simulink model "rti1401_program_controls_2018"  (R2017b)
settings: Solver=ode1  StartTime=0.0  StopTime=Inf  FixedStep=0.001  RelTol=1e-3  EnableMultiTasking=on
PreLoadFcn:
  | dataCar
  | load_vars
  | structAero
  | structEstimPar
  | structSensors
  | structSettings
PostLoadFcn:
  | , if any(exist('dsrtsu_mdlpostloadfcn', 'file') == [2, 3, 6]), try dsrtsu_mdlpostloadfcn('Execute', bdroot); catch fprintf('Error in PostLoadFcn (dsrtsu_mdlpostloadfcn) for model "%s":\n %s\n', bdroot, lasterr); end, end,
InitFcn:
  | dataCar
  | load_vars
  | structAero
  | structEstimPar
  | structSensors
  | structSettings
StartFcn:
  | dataCar
  | load_vars
  | structAero
  | structEstimPar
  | structSensors
  | structSettings
values from neighbouring files (symbols this model uses):
  Throttle_limits = [0.15, 0.90, 0.16, 0.92]    [load_vars.m]
undefined symbols (not defined in the file or in its folder): car, sensors, tau
libraries: rtican x44, hdlsllib x32, simulink x8, rti1401lib_II_base x1
(part 5 of 11)

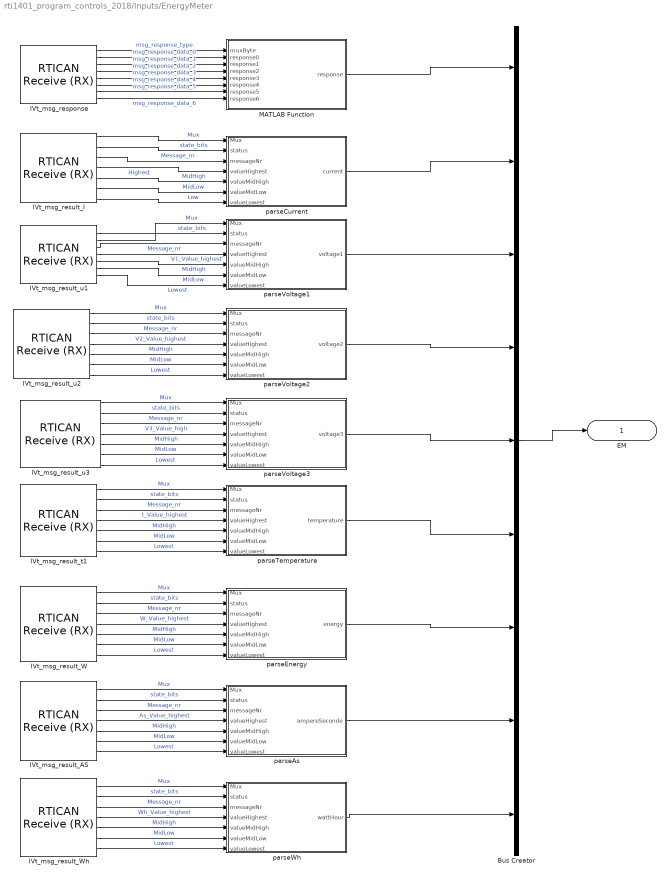
== system rti1401_program_controls_2018/Inputs/EnergyMeter ==
  Bus Creator : BusCreator  Inputs=9
  IVt_msg_response : rtican/RTICAN Receive (RX)   Reserved1=[]  Reserved2=[]  Reserved3=[]  Reserved4=[]  SfcnMessage=[]  Msg_Struct=[]  BoardTypeNo=[]  BoardNo=[]  ChannelNo=[]  Parameters=[]  DialogFcn=[]  UnitName=[]  Revision=[]  UnitValues=[]  DSProperties=struct('RTI',struct('Version',uint32(5),'BlockType',struct('isSLSource',uint8(1),'isSLSink',uint8(1),'isHWSource',uint8(0),'isHWSink',uint8(0),'isSetup',uint8(0),'isInline',uint8(1),'isNonInline',uint8(0),'isInterrupt',uint8(0),'isChannelwise',uint8(0)),'IOBoardType','RTICAN','UnitType','MESSAGE','Identifier','RX','DialogType','MSVC','BlockSet','RTICAN','SlaveProcessor','CAN'))  RTIBlockInterface=struct('OutputPortsWidth',int32([1 1 1 1 1 1 1 1]),'OutputPortsActive',[1 1 1 1 1 1 1 1],'OutputPortsName',{{'msg_response_type','msg_response_data_0','msg_response_data_1','msg_response_data_2','msg_response_data_3','msg_response_data_4','msg_response_data_5','msg_response_data_6'}},'OutputPortsDataType',{{'SS_UINT8','SS_UINT8','SS_UINT8','SS_UINT8','SS_UINT8','SS_UINT8','SS_UINT8','SS_UINT8'}},'OutputPortsLabel',{{'msg_response_type','msg_response_data_0','msg_response_data_1','msg_response_data_2','msg_response_data_3','msg_response_data_4','msg_response_data_5','msg_response_data_6'}},'OutputPortsLabelMode','ON','InputPortsWidth',int32(0),'InputPortsActive',0,'DialogFcn','rtican_message_interface_gui','BlockDisplay',{{'','center'}},'IconTransparency','on','ParameterTunableNames',{{}},'InitLevel',3,'BlockName',struct('Token',{{'IVt_msg_response'}}),'SampleTime',{{-1}},'TriggerPort',{{'none'}},'EnablePort',{{'none'}})  RTIBlockParameters=struct('BoardTypeNo',{{1,'OFF',[]}},'BoardNo',{{2,'ON',[1 16]}},'ChannelNo',{{2,'ON',[1 2]}},'Parameters',{{struct('DataFileSupport',struct('DataFileSelectedMaster',0,'DataFileSelectedLocal',0,'DataFileName',['<no datafile support>|'],'DataFileDate','','SelectedFile',['<no file selected>']),'Options',struct('StatusSelected',0,'TimeSelected',0,'DeltaTimeSelected',0,'BytePortSelected',0,'MessageLengthSelected',0,'TriggerPort',struct('Selected',0,'TriggerType',0),'UserCoding',struct('Selected',0,'InterfaceFile','UserDecodingFile','FcnName','UserDecodeFcn','InportSelected',0,'InportWidth',1,'OutportSelected',0,'OutportWidth',1),'EnablePortSelected',0,'SignalOnPortnameSelected',1,'UseRXService',0),'Message',struct('MsgOnBlocknameSelected',1,'MsgName','IVt_msg_response','MsgIdFormat',0,'MsgId',1297,'MsgLength',8,'NumSignals',8,'SampleTime',-1,'Signal',struct('SgnName',{'msg_response_type','msg_response_data_0','msg_response_data_1','msg_response_data_2','msg_response_data_3','msg_response_data_4','msg_response_data_5','msg_response_data_6'},'SgnStartBit',{0,8,16,24,32,40,48,56},'SgnLength',{8,8,8,8,8,8,8,8},'SgnType',{0,0,0,0,0,0,0,0},'ModeValue',{-1,-1,-1,-1,-1,-1,-1,-1},'DataType',{0,0,0,0,0,0,0,0},'ByteLayout',{1,1,1,1,1,1,1,1},'Factor',{1,1,1,1,1,1,1,1},'Offset',{0,0,0,0,0,0,0,0},'SgnComment',{{''},{''},{''},{''},{''},{''},{''},{''}},'SgnUnit',{'','','','','','','',''},'Min',{0,0,0,0,0,0,0,0},'Max',{255,255,255,255,255,255,255,255},'SLDataType',{'SS_UINT8','SS_UINT8','SS_UINT8','SS_UINT8','SS_UINT8','SS_UINT8','SS_UINT8','SS_UINT8'}),'MsgIdNumFormat',1,'MsgComment',{{''}}),'Version',1.2,'general',struct('isFromLib',0)),'OFF',[]}},'GroupId',{{struct('Group',{{'RTICAN'}},'No',4,'Behavior',{{'NAMECHANGE'}},'BlockType',{{'SINK'}},'NameChangeFlag',0),'OFF',[]}},'SFcnRTICANMessage',{{struct('MsgType','RX','SFcnPortType','Scalar','MsgName','IVt_msg_response','MsgIdFormat','STD','MsgId',1297,'MsgLength',8,'NumSignals',8,'SampleTime',-1,'Signal',struct('SgnName',{'msg_response_type','msg_response_data_0','msg_response_data_1','msg_response_data_2','msg_response_data_3','msg_response_data_4','msg_response_data_5','msg_response_data_6'},'SgnStartBit',{0,8,16,24,32,40,48,56},'SgnLength',{8,8,8,8,8,8,8,8},'SgnType',{'standard','standard','standard','standard','standard','standard','standard','standard'},'ModeValue',{-1,-1,-1,-1,-1,-1,-1,-1},'DataType',{['unsigned int'],['unsigned int'],['unsigned int'],['unsigned int'],['unsigned int'],['unsigned int'],['unsigned int'],['unsigned int']},'ByteLayout',{['big endian'],['big endian'],['big endian'],['big endian'],['big endian'],['big endian'],['big endian'],['big endian']},'Factor',{1,1,1,1,1,1,1,1},'Offset',{0,0,0,0,0,0,0,0},'SLDataType',{'SS_UINT8','SS_UINT8','SS_UINT8','SS_UINT8','SS_UINT8','SS_UINT8','SS_UINT8','SS_UINT8'}),'StatusSelected','no','TimeSelected','no','DeltaTimeSelected','no','BytePortSelected','no','MessageLengthSelected','no','TriggerPort',struct('Selected','no','TriggerType',0),'UserCoding',struct('Selected','no','InterfaceFile','UserDecodingFile','FcnName','UserDecodeFcn','InportSelected','no','InportWidth',1,'OutportSelected','no','OutportWidth',1),'EnablePortSelected','no','UseRXService','no','BoardType','DS1','BoardNo',2,'ControllerNo',2),'OFF',[]}},'TLCFileName',{{'rtican_rx_message','OFF',[]}})  RTISFcnParameters=struct('SFcnRTICANMessage','struct','TLCFileName','char')  RTIBlockParaDefault=struct('BoardTypeNo',4302,'BoardNo',1,'ChannelNo',1,'Parameters',struct('DataFileSupport',struct('DataFileSelectedMaster',0,'DataFileSelectedLocal',0,'DataFileName','','DataFileDate','','SelectedFile',['<no file selected>']),'Options',struct('StatusSelected',1,'TimeSelected',1,'DeltaTimeSelected',1,'BytePortSelected',0,'MessageLengthSelected',0,'TriggerPort',struct('Selected',0,'TriggerType','rising'),'UserCoding',struct('Selected',0,'InterfaceFile','UserDecodingFile','FcnName','UserDecodeFcn','InportSelected',0,'InportWidth',1,'OutportSelected',0,'OutportWidth',1),'EnablePortSelected',0,'SignalOnPortnameSelected',1,'UseRXService',0),'Message',struct('MsgOnBlocknameSelected',0,'MsgName',['RX Message'],'MsgIdFormat',0,'MsgId',100,'MsgLength',8,'NumSignals',1,'SampleTime',-1,'Signal',struct('SgnName',['RX signal'],'SgnStartBit',0,'SgnLength',8,'SgnType',0,'ModeValue',-1,'DataType',0,'SLDataType','SS_DOUBLE','ByteLayout',0,'Factor',1,'Offset',0,'Min',0,'Max',255,'SgnComment',{{}},'SgnUnit',''),'MsgIdNumFormat',0,'MsgComment',{{''}}),'Version',1.2,'general',struct('isFromLib',1)),'GroupId',struct('Group',{{'RTICAN'}},'No',1,'Behavior',{{'NAMECHANGE'}},'BlockType',{{'SINK'}},'NameChangeFlag',0),'SFcnRTICANMessage',struct('MsgType','RX','MsgName',['RX Message'],'MsgIdFormat','STD','MsgId',100,'MsgLength',8,'NumSignals',1,'SampleTime',-1,'Signal',struct('SgnName',['RX signal'],'SgnStartBit',0,'SgnLength',8,'SgnType','standard','ModeValue',-1,'DataType',['unsigned int'],'ByteLayout',['little endian'],'SLDataType','SS_DOUBLE','Factor',1,'Offset',0),'StatusSelected','yes','TimeSelected','yes','DeltaTimeSelected','yes','BytePortSelected','no','MessageLengthSelected','no','EnablePortSelected','no','UserCoding',struct('Selected','no','InterfaceFile','UserDecodingFile','FcnName','UserDecodeFcn','InportSelected','no','InportWidth',1,'OutportSelected','no','OutportWidth',1),'TriggerPort',struct('Selected','no','TriggerType','rising'),'UseRXService','no','BoardType','DS4302','BoardNo',1,'ControllerNo',1,'SFcnPortType','Scalar'),'TLCFileName','rtican_rx_message')
      settings: AttributesFormatString=Group Id: RTICAN4\n
  IVt_msg_result_AS : rtican/RTICAN Receive (RX)   Reserved1=[]  Reserved2=[]  Reserved3=[]  Reserved4=[]  SfcnMessage=[]  Msg_Struct=[]  BoardTypeNo=[]  BoardNo=[]  ChannelNo=[]  Parameters=[]  DialogFcn=[]  UnitName=[]  Revision=[]  UnitValues=[]  DSProperties=struct('RTI',struct('Version',uint32(5),'BlockType',struct('isSLSource',uint8(1),'isSLSink',uint8(1),'isHWSource',uint8(0),'isHWSink',uint8(0),'isSetup',uint8(0),'isInline',uint8(1),'isNonInline',uint8(0),'isInterrupt',uint8(0),'isChannelwise',uint8(0)),'IOBoardType','RTICAN','UnitType','MESSAGE','Identifier','RX','DialogType','MSVC','BlockSet','RTICAN','SlaveProcessor','CAN'))  RTIBlockInterface=struct('OutputPortsWidth',int32([1 1 1 1 1 1 1]),'OutputPortsActive',[1 1 1 1 1 1 1],'OutputPortsName',{{'Mux','state_bits','Message_nr','As_Value_highest','MidHigh','MidLow','Lowest'}},'OutputPortsDataType',{{'SS_UINT8','SS_UINT8','SS_UINT8','SS_UINT8','SS_UINT8','SS_UINT8','SS_UINT8'}},'OutputPortsLabel',{{'Mux','state_bits','Message_nr','As_Value_highest','MidHigh','MidLow','Lowest'}},'OutputPortsLabelMode','ON','InputPortsWidth',int32(0),'InputPortsActive',0,'DialogFcn','rtican_message_interface_gui','BlockDisplay',{{'','center'}},'IconTransparency','on','ParameterTunableNames',{{}},'InitLevel',3,'BlockName',struct('Token',{{'IVt_msg_result_AS'}}),'SampleTime',{{-1}},'TriggerPort',{{'none'}},'EnablePort',{{'none'}})  RTIBlockParameters=struct('BoardTypeNo',{{1,'OFF',[]}},'BoardNo',{{2,'ON',[1 16]}},'ChannelNo',{{2,'ON',[1 2]}},'Parameters',{{struct('DataFileSupport',struct('DataFileSelectedMaster',0,'DataFileSelectedLocal',0,'DataFileName',['<no datafile support>|'],'DataFileDate','','SelectedFile',['<no file selected>']),'Options',struct('StatusSelected',0,'TimeSelected',0,'DeltaTimeSelected',0,'BytePortSelected',0,'MessageLengthSelected',0,'TriggerPort',struct('Selected',0,'TriggerType',0),'UserCoding',struct('Selected',0,'InterfaceFile','UserDecodingFile','FcnName','UserDecodeFcn','InportSelected',0,'InportWidth',1,'OutportSelected',0,'OutportWidth',1),'EnablePortSelected',0,'SignalOnPortnameSelected',1,'UseRXService',0),'Message',struct('MsgOnBlocknameSelected',1,'MsgName','IVt_msg_result_AS','MsgIdFormat',0,'MsgId',1319,'MsgLength',6,'NumSignals',7,'SampleTime',-1,'Signal',struct('SgnName',{'Mux','state_bits','Message_nr','As_Value_highest','MidHigh','MidLow','Lowest'},'SgnStartBit',{0,8,12,16,24,32,40},'SgnLength',{8,4,4,8,8,8,8},'SgnType',{0,0,0,0,0,0,0},'ModeValue',{-1,-1,-1,-1,-1,-1,-1},'DataType',{0,0,0,0,0,0,0},'ByteLayout',{1,1,1,1,1,1,1},'Factor',{1,1,1,1,1,1,1},'Offset',{0,0,0,0,0,0,0},'SgnComment',{{''},{''},{''},{''},{''},{''},{''}},'SgnUnit',{'','','','','','',''},'Min',{0,0,0,0,0,0,0},'Max',{255,255,255,255,255,255,255},'SLDataType',{'SS_UINT8','SS_UINT8','SS_UINT8','SS_UINT8','SS_UINT8','SS_UINT8','SS_UINT8'}),'MsgIdNumFormat',1,'MsgComment',{{''}}),'Version',1.2,'general',struct('isFromLib',0)),'OFF',[]}},'GroupId',{{struct('Group',{{'RTICAN'}},'No',4,'Behavior',{{'NAMECHANGE'}},'BlockType',{{'SINK'}},'NameChangeFlag',0),'OFF',[]}},'SFcnRTICANMessage',{{struct('MsgType','RX','SFcnPortType','Scalar','MsgName','IVt_msg_result_AS','MsgIdFormat','STD','MsgId',1319,'MsgLength',6,'NumSignals',7,'SampleTime',-1,'Signal',struct('SgnName',{'Mux','state_bits','Message_nr','As_Value_highest','MidHigh','MidLow','Lowest'},'SgnStartBit',{0,8,12,16,24,32,40},'SgnLength',{8,4,4,8,8,8,8},'SgnType',{'standard','standard','standard','standard','standard','standard','standard'},'ModeValue',{-1,-1,-1,-1,-1,-1,-1},'DataType',{['unsigned int'],['unsigned int'],['unsigned int'],['unsigned int'],['unsigned int'],['unsigned int'],['unsigned int']},'ByteLayout',{['big endian'],['big endian'],['big endian'],['big endian'],['big endian'],['big endian'],['big endian']},'Factor',{1,1,1,1,1,1,1},'Offset',{0,0,0,0,0,0,0},'SLDataType',{'SS_UINT8','SS_UINT8','SS_UINT8','SS_UINT8','SS_UINT8','SS_UINT8','SS_UINT8'}),'StatusSelected','no','TimeSelected','no','DeltaTimeSelected','no','BytePortSelected','no','MessageLengthSelected','no','TriggerPort',struct('Selected','no','TriggerType',0),'UserCoding',struct('Selected','no','InterfaceFile','UserDecodingFile','FcnName','UserDecodeFcn','InportSelected','no','InportWidth',1,'OutportSelected','no','OutportWidth',1),'EnablePortSelected','no','UseRXService','no','BoardType','DS1','BoardNo',2,'ControllerNo',2),'OFF',[]}},'TLCFileName',{{'rtican_rx_message','OFF',[]}})  RTISFcnParameters=struct('SFcnRTICANMessage','struct','TLCFileName','char')  RTIBlockParaDefault=struct('BoardTypeNo',4302,'BoardNo',1,'ChannelNo',1,'Parameters',struct('DataFileSupport',struct('DataFileSelectedMaster',0,'DataFileSelectedLocal',0,'DataFileName','','DataFileDate','','SelectedFile',['<no file selected>']),'Options',struct('StatusSelected',1,'TimeSelected',1,'DeltaTimeSelected',1,'BytePortSelected',0,'MessageLengthSelected',0,'TriggerPort',struct('Selected',0,'TriggerType','rising'),'UserCoding',struct('Selected',0,'InterfaceFile','UserDecodingFile','FcnName','UserDecodeFcn','InportSelected',0,'InportWidth',1,'OutportSelected',0,'OutportWidth',1),'EnablePortSelected',0,'SignalOnPortnameSelected',1,'UseRXService',0),'Message',struct('MsgOnBlocknameSelected',0,'MsgName',['RX Message'],'MsgIdFormat',0,'MsgId',100,'MsgLength',8,'NumSignals',1,'SampleTime',-1,'Signal',struct('SgnName',['RX signal'],'SgnStartBit',0,'SgnLength',8,'SgnType',0,'ModeValue',-1,'DataType',0,'SLDataType','SS_DOUBLE','ByteLayout',0,'Factor',1,'Offset',0,'Min',0,'Max',255,'SgnComment',{{}},'SgnUnit',''),'MsgIdNumFormat',0,'MsgComment',{{''}}),'Version',1.2,'general',struct('isFromLib',1)),'GroupId',struct('Group',{{'RTICAN'}},'No',1,'Behavior',{{'NAMECHANGE'}},'BlockType',{{'SINK'}},'NameChangeFlag',0),'SFcnRTICANMessage',struct('MsgType','RX','MsgName',['RX Message'],'MsgIdFormat','STD','MsgId',100,'MsgLength',8,'NumSignals',1,'SampleTime',-1,'Signal',struct('SgnName',['RX signal'],'SgnStartBit',0,'SgnLength',8,'SgnType','standard','ModeValue',-1,'DataType',['unsigned int'],'ByteLayout',['little endian'],'SLDataType','SS_DOUBLE','Factor',1,'Offset',0),'StatusSelected','yes','TimeSelected','yes','DeltaTimeSelected','yes','BytePortSelected','no','MessageLengthSelected','no','EnablePortSelected','no','UserCoding',struct('Selected','no','InterfaceFile','UserDecodingFile','FcnName','UserDecodeFcn','InportSelected','no','InportWidth',1,'OutportSelected','no','OutportWidth',1),'TriggerPort',struct('Selected','no','TriggerType','rising'),'UseRXService','no','BoardType','DS4302','BoardNo',1,'ControllerNo',1,'SFcnPortType','Scalar'),'TLCFileName','rtican_rx_message')
      settings: AttributesFormatString=Group Id: RTICAN4\n
  IVt_msg_result_I : rtican/RTICAN Receive (RX)   Reserved1=[]  Reserved2=[]  Reserved3=[]  Reserved4=[]  SfcnMessage=[]  Msg_Struct=[]  BoardTypeNo=[]  BoardNo=[]  ChannelNo=[]  Parameters=[]  DialogFcn=[]  UnitName=[]  Revision=[]  UnitValues=[]  DSProperties=struct('RTI',struct('Version',uint32(5),'BlockType',struct('isSLSource',uint8(1),'isSLSink',uint8(1),'isHWSource',uint8(0),'isHWSink',uint8(0),'isSetup',uint8(0),'isInline',uint8(1),'isNonInline',uint8(0),'isInterrupt',uint8(0),'isChannelwise',uint8(0)),'IOBoardType','RTICAN','UnitType','MESSAGE','Identifier','RX','DialogType','MSVC','BlockSet','RTICAN','SlaveProcessor','CAN'))  RTIBlockInterface=struct('OutputPortsWidth',int32([1 1 1 1 1 1 1]),'OutputPortsActive',[1 1 1 1 1 1 1],'OutputPortsName',{{'Mux','state_bits','Message_nr','Highest','MidHigh','MidLow','Low'}},'OutputPortsDataType',{{'SS_UINT8','SS_UINT8','SS_UINT8','SS_UINT8','SS_UINT8','SS_UINT8','SS_UINT8'}},'OutputPortsLabel',{{'Mux','state_bits','Message_nr','Highest','MidHigh','MidLow','Low'}},'OutputPortsLabelMode','ON','InputPortsWidth',int32(0),'InputPortsActive',0,'DialogFcn','rtican_message_interface_gui','BlockDisplay',{{'','center'}},'IconTransparency','on','ParameterTunableNames',{{}},'InitLevel',3,'BlockName',struct('Token',{{'IVt_msg_result_I'}}),'SampleTime',{{-1}},'TriggerPort',{{'none'}},'EnablePort',{{'none'}})  RTIBlockParameters=struct('BoardTypeNo',{{1,'OFF',[]}},'BoardNo',{{2,'ON',[1 16]}},'ChannelNo',{{2,'ON',[1 2]}},'Parameters',{{struct('DataFileSupport',struct('DataFileSelectedMaster',0,'DataFileSelectedLocal',0,'DataFileName',['<no datafile support>|'],'DataFileDate','','SelectedFile',['<no file selected>']),'Options',struct('StatusSelected',0,'TimeSelected',0,'DeltaTimeSelected',0,'BytePortSelected',0,'MessageLengthSelected',0,'TriggerPort',struct('Selected',0,'TriggerType',0),'UserCoding',struct('Selected',0,'InterfaceFile','UserDecodingFile','FcnName','UserDecodeFcn','InportSelected',0,'InportWidth',1,'OutportSelected',0,'OutportWidth',1),'EnablePortSelected',0,'SignalOnPortnameSelected',1,'UseRXService',0),'Message',struct('MsgOnBlocknameSelected',1,'MsgName','IVt_msg_result_I','MsgIdFormat',0,'MsgId',1313,'MsgLength',6,'NumSignals',7,'SampleTime',-1,'Signal',struct('SgnName',{'Mux','state_bits','Message_nr','Highest','MidHigh','MidLow','Low'},'SgnStartBit',{0,8,12,16,24,32,40},'SgnLength',{8,4,4,8,8,8,8},'SgnType',{0,0,0,0,0,0,0},'ModeValue',{-1,-1,-1,-1,-1,-1,-1},'DataType',{0,0,0,0,0,0,0},'ByteLayout',{1,1,1,1,1,1,1},'Factor',{1,1,1,1,1,1,1},'Offset',{0,0,0,0,0,0,0},'SgnComment',{{''},{''},{''},{''},{''},{''},{''}},'SgnUnit',{'','','','','','',''},'Min',{0,0,0,0,0,0,0},'Max',{255,255,255,0,0,0,0},'SLDataType',{'SS_UINT8','SS_UINT8','SS_UINT8','SS_UINT8','SS_UINT8','SS_UINT8','SS_UINT8'}),'MsgIdNumFormat',1,'MsgComment',{{''}}),'Version',1.2,'general',struct('isFromLib',0)),'OFF',[]}},'GroupId',{{struct('Group',{{'RTICAN'}},'No',4,'Behavior',{{'NAMECHANGE'}},'BlockType',{{'SINK'}},'NameChangeFlag',0),'OFF',[]}},'SFcnRTICANMessage',{{struct('MsgType','RX','SFcnPortType','Scalar','MsgName','IVt_msg_result_I','MsgIdFormat','STD','MsgId',1313,'MsgLength',6,'NumSignals',7,'SampleTime',-1,'Signal',struct('SgnName',{'Mux','state_bits','Message_nr','Highest','MidHigh','MidLow','Low'},'SgnStartBit',{0,8,12,16,24,32,40},'SgnLength',{8,4,4,8,8,8,8},'SgnType',{'standard','standard','standard','standard','standard','standard','standard'},'ModeValue',{-1,-1,-1,-1,-1,-1,-1},'DataType',{['unsigned int'],['unsigned int'],['unsigned int'],['unsigned int'],['unsigned int'],['unsigned int'],['unsigned int']},'ByteLayout',{['big endian'],['big endian'],['big endian'],['big endian'],['big endian'],['big endian'],['big endian']},'Factor',{1,1,1,1,1,1,1},'Offset',{0,0,0,0,0,0,0},'SLDataType',{'SS_UINT8','SS_UINT8','SS_UINT8','SS_UINT8','SS_UINT8','SS_UINT8','SS_UINT8'}),'StatusSelected','no','TimeSelected','no','DeltaTimeSelected','no','BytePortSelected','no','MessageLengthSelected','no','TriggerPort',struct('Selected','no','TriggerType',0),'UserCoding',struct('Selected','no','InterfaceFile','UserDecodingFile','FcnName','UserDecodeFcn','InportSelected','no','InportWidth',1,'OutportSelected','no','OutportWidth',1),'EnablePortSelected','no','UseRXService','no','BoardType','DS1','BoardNo',2,'ControllerNo',2),'OFF',[]}},'TLCFileName',{{'rtican_rx_message','OFF',[]}})  RTISFcnParameters=struct('SFcnRTICANMessage','struct','TLCFileName','char')  RTIBlockParaDefault=struct('BoardTypeNo',4302,'BoardNo',1,'ChannelNo',1,'Parameters',struct('DataFileSupport',struct('DataFileSelectedMaster',0,'DataFileSelectedLocal',0,'DataFileName','','DataFileDate','','SelectedFile',['<no file selected>']),'Options',struct('StatusSelected',1,'TimeSelected',1,'DeltaTimeSelected',1,'BytePortSelected',0,'MessageLengthSelected',0,'TriggerPort',struct('Selected',0,'TriggerType','rising'),'UserCoding',struct('Selected',0,'InterfaceFile','UserDecodingFile','FcnName','UserDecodeFcn','InportSelected',0,'InportWidth',1,'OutportSelected',0,'OutportWidth',1),'EnablePortSelected',0,'SignalOnPortnameSelected',1,'UseRXService',0),'Message',struct('MsgOnBlocknameSelected',0,'MsgName',['RX Message'],'MsgIdFormat',0,'MsgId',100,'MsgLength',8,'NumSignals',1,'SampleTime',-1,'Signal',struct('SgnName',['RX signal'],'SgnStartBit',0,'SgnLength',8,'SgnType',0,'ModeValue',-1,'DataType',0,'SLDataType','SS_DOUBLE','ByteLayout',0,'Factor',1,'Offset',0,'Min',0,'Max',255,'SgnComment',{{}},'SgnUnit',''),'MsgIdNumFormat',0,'MsgComment',{{''}}),'Version',1.2,'general',struct('isFromLib',1)),'GroupId',struct('Group',{{'RTICAN'}},'No',1,'Behavior',{{'NAMECHANGE'}},'BlockType',{{'SINK'}},'NameChangeFlag',0),'SFcnRTICANMessage',struct('MsgType','RX','MsgName',['RX Message'],'MsgIdFormat','STD','MsgId',100,'MsgLength',8,'NumSignals',1,'SampleTime',-1,'Signal',struct('SgnName',['RX signal'],'SgnStartBit',0,'SgnLength',8,'SgnType','standard','ModeValue',-1,'DataType',['unsigned int'],'ByteLayout',['little endian'],'SLDataType','SS_DOUBLE','Factor',1,'Offset',0),'StatusSelected','yes','TimeSelected','yes','DeltaTimeSelected','yes','BytePortSelected','no','MessageLengthSelected','no','EnablePortSelected','no','UserCoding',struct('Selected','no','InterfaceFile','UserDecodingFile','FcnName','UserDecodeFcn','InportSelected','no','InportWidth',1,'OutportSelected','no','OutportWidth',1),'TriggerPort',struct('Selected','no','TriggerType','rising'),'UseRXService','no','BoardType','DS4302','BoardNo',1,'ControllerNo',1,'SFcnPortType','Scalar'),'TLCFileName','rtican_rx_message')
      settings: AttributesFormatString=Group Id: RTICAN4\n
  IVt_msg_result_W : rtican/RTICAN Receive (RX)   Reserved1=[]  Reserved2=[]  Reserved3=[]  Reserved4=[]  SfcnMessage=[]  Msg_Struct=[]  BoardTypeNo=[]  BoardNo=[]  ChannelNo=[]  Parameters=[]  DialogFcn=[]  UnitName=[]  Revision=[]  UnitValues=[]  DSProperties=struct('RTI',struct('Version',uint32(5),'BlockType',struct('isSLSource',uint8(1),'isSLSink',uint8(1),'isHWSource',uint8(0),'isHWSink',uint8(0),'isSetup',uint8(0),'isInline',uint8(1),'isNonInline',uint8(0),'isInterrupt',uint8(0),'isChannelwise',uint8(0)),'IOBoardType','RTICAN','UnitType','MESSAGE','Identifier','RX','DialogType','MSVC','BlockSet','RTICAN','SlaveProcessor','CAN'))  RTIBlockInterface=struct('OutputPortsWidth',int32([1 1 1 1 1 1 1]),'OutputPortsActive',[1 1 1 1 1 1 1],'OutputPortsName',{{'Mux','state_bits','Message_nr','W_Value_highest','MidHigh','MidLow','Lowest'}},'OutputPortsDataType',{{'SS_UINT8','SS_UINT8','SS_UINT8','SS_UINT8','SS_UINT8','SS_UINT8','SS_UINT8'}},'OutputPortsLabel',{{'Mux','state_bits','Message_nr','W_Value_highest','MidHigh','MidLow','Lowest'}},'OutputPortsLabelMode','ON','InputPortsWidth',int32(0),'InputPortsActive',0,'DialogFcn','rtican_message_interface_gui','BlockDisplay',{{'','center'}},'IconTransparency','on','ParameterTunableNames',{{}},'InitLevel',3,'BlockName',struct('Token',{{'IVt_msg_result_W'}}),'SampleTime',{{-1}},'TriggerPort',{{'none'}},'EnablePort',{{'none'}})  RTIBlockParameters=struct('BoardTypeNo',{{1,'OFF',[]}},'BoardNo',{{2,'ON',[1 16]}},'ChannelNo',{{2,'ON',[1 2]}},'Parameters',{{struct('DataFileSupport',struct('DataFileSelectedMaster',0,'DataFileSelectedLocal',0,'DataFileName',['<no datafile support>|'],'DataFileDate','','SelectedFile',['<no file selected>']),'Options',struct('StatusSelected',0,'TimeSelected',0,'DeltaTimeSelected',0,'BytePortSelected',0,'MessageLengthSelected',0,'TriggerPort',struct('Selected',0,'TriggerType',0),'UserCoding',struct('Selected',0,'InterfaceFile','UserDecodingFile','FcnName','UserDecodeFcn','InportSelected',0,'InportWidth',1,'OutportSelected',0,'OutportWidth',1),'EnablePortSelected',0,'SignalOnPortnameSelected',1,'UseRXService',0),'Message',struct('MsgOnBlocknameSelected',1,'MsgName','IVt_msg_result_W','MsgIdFormat',0,'MsgId',1318,'MsgLength',6,'NumSignals',7,'SampleTime',-1,'Signal',struct('SgnName',{'Mux','state_bits','Message_nr','W_Value_highest','MidHigh','MidLow','Lowest'},'SgnStartBit',{0,8,12,16,24,32,40},'SgnLength',{8,4,4,8,8,8,8},'SgnType',{0,0,0,0,0,0,0},'ModeValue',{-1,-1,-1,-1,-1,-1,-1},'DataType',{0,0,0,0,0,0,0},'ByteLayout',{1,1,1,1,1,1,1},'Factor',{1,1,1,1,1,1,1},'Offset',{0,0,0,0,0,0,0},'SgnComment',{{''},{''},{''},{''},{''},{''},{''}},'SgnUnit',{'','','','','','',''},'Min',{0,0,0,0,0,0,0},'Max',{255,255,255,255,255,255,255},'SLDataType',{'SS_UINT8','SS_UINT8','SS_UINT8','SS_UINT8','SS_UINT8','SS_UINT8','SS_UINT8'}),'MsgIdNumFormat',1,'MsgComment',{{''}}),'Version',1.2,'general',struct('isFromLib',0)),'OFF',[]}},'GroupId',{{struct('Group',{{'RTICAN'}},'No',4,'Behavior',{{'NAMECHANGE'}},'BlockType',{{'SINK'}},'NameChangeFlag',0),'OFF',[]}},'SFcnRTICANMessage',{{struct('MsgType','RX','SFcnPortType','Scalar','MsgName','IVt_msg_result_W','MsgIdFormat','STD','MsgId',1318,'MsgLength',6,'NumSignals',7,'SampleTime',-1,'Signal',struct('SgnName',{'Mux','state_bits','Message_nr','W_Value_highest','MidHigh','MidLow','Lowest'},'SgnStartBit',{0,8,12,16,24,32,40},'SgnLength',{8,4,4,8,8,8,8},'SgnType',{'standard','standard','standard','standard','standard','standard','standard'},'ModeValue',{-1,-1,-1,-1,-1,-1,-1},'DataType',{['unsigned int'],['unsigned int'],['unsigned int'],['unsigned int'],['unsigned int'],['unsigned int'],['unsigned int']},'ByteLayout',{['big endian'],['big endian'],['big endian'],['big endian'],['big endian'],['big endian'],['big endian']},'Factor',{1,1,1,1,1,1,1},'Offset',{0,0,0,0,0,0,0},'SLDataType',{'SS_UINT8','SS_UINT8','SS_UINT8','SS_UINT8','SS_UINT8','SS_UINT8','SS_UINT8'}),'StatusSelected','no','TimeSelected','no','DeltaTimeSelected','no','BytePortSelected','no','MessageLengthSelected','no','TriggerPort',struct('Selected','no','TriggerType',0),'UserCoding',struct('Selected','no','InterfaceFile','UserDecodingFile','FcnName','UserDecodeFcn','InportSelected','no','InportWidth',1,'OutportSelected','no','OutportWidth',1),'EnablePortSelected','no','UseRXService','no','BoardType','DS1','BoardNo',2,'ControllerNo',2),'OFF',[]}},'TLCFileName',{{'rtican_rx_message','OFF',[]}})  RTISFcnParameters=struct('SFcnRTICANMessage','struct','TLCFileName','char')  RTIBlockParaDefault=struct('BoardTypeNo',4302,'BoardNo',1,'ChannelNo',1,'Parameters',struct('DataFileSupport',struct('DataFileSelectedMaster',0,'DataFileSelectedLocal',0,'DataFileName','','DataFileDate','','SelectedFile',['<no file selected>']),'Options',struct('StatusSelected',1,'TimeSelected',1,'DeltaTimeSelected',1,'BytePortSelected',0,'MessageLengthSelected',0,'TriggerPort',struct('Selected',0,'TriggerType','rising'),'UserCoding',struct('Selected',0,'InterfaceFile','UserDecodingFile','FcnName','UserDecodeFcn','InportSelected',0,'InportWidth',1,'OutportSelected',0,'OutportWidth',1),'EnablePortSelected',0,'SignalOnPortnameSelected',1,'UseRXService',0),'Message',struct('MsgOnBlocknameSelected',0,'MsgName',['RX Message'],'MsgIdFormat',0,'MsgId',100,'MsgLength',8,'NumSignals',1,'SampleTime',-1,'Signal',struct('SgnName',['RX signal'],'SgnStartBit',0,'SgnLength',8,'SgnType',0,'ModeValue',-1,'DataType',0,'SLDataType','SS_DOUBLE','ByteLayout',0,'Factor',1,'Offset',0,'Min',0,'Max',255,'SgnComment',{{}},'SgnUnit',''),'MsgIdNumFormat',0,'MsgComment',{{''}}),'Version',1.2,'general',struct('isFromLib',1)),'GroupId',struct('Group',{{'RTICAN'}},'No',1,'Behavior',{{'NAMECHANGE'}},'BlockType',{{'SINK'}},'NameChangeFlag',0),'SFcnRTICANMessage',struct('MsgType','RX','MsgName',['RX Message'],'MsgIdFormat','STD','MsgId',100,'MsgLength',8,'NumSignals',1,'SampleTime',-1,'Signal',struct('SgnName',['RX signal'],'SgnStartBit',0,'SgnLength',8,'SgnType','standard','ModeValue',-1,'DataType',['unsigned int'],'ByteLayout',['little endian'],'SLDataType','SS_DOUBLE','Factor',1,'Offset',0),'StatusSelected','yes','TimeSelected','yes','DeltaTimeSelected','yes','BytePortSelected','no','MessageLengthSelected','no','EnablePortSelected','no','UserCoding',struct('Selected','no','InterfaceFile','UserDecodingFile','FcnName','UserDecodeFcn','InportSelected','no','InportWidth',1,'OutportSelected','no','OutportWidth',1),'TriggerPort',struct('Selected','no','TriggerType','rising'),'UseRXService','no','BoardType','DS4302','BoardNo',1,'ControllerNo',1,'SFcnPortType','Scalar'),'TLCFileName','rtican_rx_message')
      settings: AttributesFormatString=Group Id: RTICAN4\n
  IVt_msg_result_Wh : rtican/RTICAN Receive (RX)   Reserved1=[]  Reserved2=[]  Reserved3=[]  Reserved4=[]  SfcnMessage=[]  Msg_Struct=[]  BoardTypeNo=[]  BoardNo=[]  ChannelNo=[]  Parameters=[]  DialogFcn=[]  UnitName=[]  Revision=[]  UnitValues=[]  DSProperties=struct('RTI',struct('Version',uint32(5),'BlockType',struct('isSLSource',uint8(1),'isSLSink',uint8(1),'isHWSource',uint8(0),'isHWSink',uint8(0),'isSetup',uint8(0),'isInline',uint8(1),'isNonInline',uint8(0),'isInterrupt',uint8(0),'isChannelwise',uint8(0)),'IOBoardType','RTICAN','UnitType','MESSAGE','Identifier','RX','DialogType','MSVC','BlockSet','RTICAN','SlaveProcessor','CAN'))  RTIBlockInterface=struct('OutputPortsWidth',int32([1 1 1 1 1 1 1]),'OutputPortsActive',[1 1 1 1 1 1 1],'OutputPortsName',{{'Mux','state_bits','Message_nr','Wh_Value_highest','MidHigh','MidLow','Lowest'}},'OutputPortsDataType',{{'SS_UINT8','SS_UINT8','SS_UINT8','SS_UINT8','SS_UINT8','SS_UINT8','SS_UINT8'}},'OutputPortsLabel',{{'Mux','state_bits','Message_nr','Wh_Value_highest','MidHigh','MidLow','Lowest'}},'OutputPortsLabelMode','ON','InputPortsWidth',int32(0),'InputPortsActive',0,'DialogFcn','rtican_message_interface_gui','BlockDisplay',{{'','center'}},'IconTransparency','on','ParameterTunableNames',{{}},'InitLevel',3,'BlockName',struct('Token',{{'IVt_msg_result_Wh'}}),'SampleTime',{{-1}},'TriggerPort',{{'none'}},'EnablePort',{{'none'}})  RTIBlockParameters=struct('BoardTypeNo',{{1,'OFF',[]}},'BoardNo',{{2,'ON',[1 16]}},'ChannelNo',{{2,'ON',[1 2]}},'Parameters',{{struct('DataFileSupport',struct('DataFileSelectedMaster',0,'DataFileSelectedLocal',0,'DataFileName',['<no datafile support>|'],'DataFileDate','','SelectedFile',['<no file selected>']),'Options',struct('StatusSelected',0,'TimeSelected',0,'DeltaTimeSelected',0,'BytePortSelected',0,'MessageLengthSelected',0,'TriggerPort',struct('Selected',0,'TriggerType',0),'UserCoding',struct('Selected',0,'InterfaceFile','UserDecodingFile','FcnName','UserDecodeFcn','InportSelected',0,'InportWidth',1,'OutportSelected',0,'OutportWidth',1),'EnablePortSelected',0,'SignalOnPortnameSelected',1,'UseRXService',0),'Message',struct('MsgOnBlocknameSelected',1,'MsgName','IVt_msg_result_Wh','MsgIdFormat',0,'MsgId',1320,'MsgLength',6,'NumSignals',7,'SampleTime',-1,'Signal',struct('SgnName',{'Mux','state_bits','Message_nr','Wh_Value_highest','MidHigh','MidLow','Lowest'},'SgnStartBit',{0,8,12,16,24,32,40},'SgnLength',{8,4,4,8,8,8,8},'SgnType',{0,0,0,0,0,0,0},'ModeValue',{-1,-1,-1,-1,-1,-1,-1},'DataType',{0,0,0,0,0,0,0},'ByteLayout',{1,1,1,1,1,1,1},'Factor',{1,1,1,1,1,1,1},'Offset',{0,0,0,0,0,0,0},'SgnComment',{{''},{''},{''},{''},{''},{''},{''}},'SgnUnit',{'','','','','','',''},'Min',{0,0,0,0,0,0,0},'Max',{255,255,255,255,255,255,255},'SLDataType',{'SS_UINT8','SS_UINT8','SS_UINT8','SS_UINT8','SS_UINT8','SS_UINT8','SS_UINT8'}),'MsgIdNumFormat',1,'MsgComment',{{''}}),'Version',1.2,'general',struct('isFromLib',0)),'OFF',[]}},'GroupId',{{struct('Group',{{'RTICAN'}},'No',4,'Behavior',{{'NAMECHANGE'}},'BlockType',{{'SINK'}},'NameChangeFlag',0),'OFF',[]}},'SFcnRTICANMessage',{{struct('MsgType','RX','SFcnPortType','Scalar','MsgName','IVt_msg_result_Wh','MsgIdFormat','STD','MsgId',1320,'MsgLength',6,'NumSignals',7,'SampleTime',-1,'Signal',struct('SgnName',{'Mux','state_bits','Message_nr','Wh_Value_highest','MidHigh','MidLow','Lowest'},'SgnStartBit',{0,8,12,16,24,32,40},'SgnLength',{8,4,4,8,8,8,8},'SgnType',{'standard','standard','standard','standard','standard','standard','standard'},'ModeValue',{-1,-1,-1,-1,-1,-1,-1},'DataType',{['unsigned int'],['unsigned int'],['unsigned int'],['unsigned int'],['unsigned int'],['unsigned int'],['unsigned int']},'ByteLayout',{['big endian'],['big endian'],['big endian'],['big endian'],['big endian'],['big endian'],['big endian']},'Factor',{1,1,1,1,1,1,1},'Offset',{0,0,0,0,0,0,0},'SLDataType',{'SS_UINT8','SS_UINT8','SS_UINT8','SS_UINT8','SS_UINT8','SS_UINT8','SS_UINT8'}),'StatusSelected','no','TimeSelected','no','DeltaTimeSelected','no','BytePortSelected','no','MessageLengthSelected','no','TriggerPort',struct('Selected','no','TriggerType',0),'UserCoding',struct('Selected','no','InterfaceFile','UserDecodingFile','FcnName','UserDecodeFcn','InportSelected','no','InportWidth',1,'OutportSelected','no','OutportWidth',1),'EnablePortSelected','no','UseRXService','no','BoardType','DS1','BoardNo',2,'ControllerNo',2),'OFF',[]}},'TLCFileName',{{'rtican_rx_message','OFF',[]}})  RTISFcnParameters=struct('SFcnRTICANMessage','struct','TLCFileName','char')  RTIBlockParaDefault=struct('BoardTypeNo',4302,'BoardNo',1,'ChannelNo',1,'Parameters',struct('DataFileSupport',struct('DataFileSelectedMaster',0,'DataFileSelectedLocal',0,'DataFileName','','DataFileDate','','SelectedFile',['<no file selected>']),'Options',struct('StatusSelected',1,'TimeSelected',1,'DeltaTimeSelected',1,'BytePortSelected',0,'MessageLengthSelected',0,'TriggerPort',struct('Selected',0,'TriggerType','rising'),'UserCoding',struct('Selected',0,'InterfaceFile','UserDecodingFile','FcnName','UserDecodeFcn','InportSelected',0,'InportWidth',1,'OutportSelected',0,'OutportWidth',1),'EnablePortSelected',0,'SignalOnPortnameSelected',1,'UseRXService',0),'Message',struct('MsgOnBlocknameSelected',0,'MsgName',['RX Message'],'MsgIdFormat',0,'MsgId',100,'MsgLength',8,'NumSignals',1,'SampleTime',-1,'Signal',struct('SgnName',['RX signal'],'SgnStartBit',0,'SgnLength',8,'SgnType',0,'ModeValue',-1,'DataType',0,'SLDataType','SS_DOUBLE','ByteLayout',0,'Factor',1,'Offset',0,'Min',0,'Max',255,'SgnComment',{{}},'SgnUnit',''),'MsgIdNumFormat',0,'MsgComment',{{''}}),'Version',1.2,'general',struct('isFromLib',1)),'GroupId',struct('Group',{{'RTICAN'}},'No',1,'Behavior',{{'NAMECHANGE'}},'BlockType',{{'SINK'}},'NameChangeFlag',0),'SFcnRTICANMessage',struct('MsgType','RX','MsgName',['RX Message'],'MsgIdFormat','STD','MsgId',100,'MsgLength',8,'NumSignals',1,'SampleTime',-1,'Signal',struct('SgnName',['RX signal'],'SgnStartBit',0,'SgnLength',8,'SgnType','standard','ModeValue',-1,'DataType',['unsigned int'],'ByteLayout',['little endian'],'SLDataType','SS_DOUBLE','Factor',1,'Offset',0),'StatusSelected','yes','TimeSelected','yes','DeltaTimeSelected','yes','BytePortSelected','no','MessageLengthSelected','no','EnablePortSelected','no','UserCoding',struct('Selected','no','InterfaceFile','UserDecodingFile','FcnName','UserDecodeFcn','InportSelected','no','InportWidth',1,'OutportSelected','no','OutportWidth',1),'TriggerPort',struct('Selected','no','TriggerType','rising'),'UseRXService','no','BoardType','DS4302','BoardNo',1,'ControllerNo',1,'SFcnPortType','Scalar'),'TLCFileName','rtican_rx_message')
      settings: AttributesFormatString=Group Id: RTICAN4\n
  IVt_msg_result_t1 : rtican/RTICAN Receive (RX)   Reserved1=[]  Reserved2=[]  Reserved3=[]  Reserved4=[]  SfcnMessage=[]  Msg_Struct=[]  BoardTypeNo=[]  BoardNo=[]  ChannelNo=[]  Parameters=[]  DialogFcn=[]  UnitName=[]  Revision=[]  UnitValues=[]  DSProperties=struct('RTI',struct('Version',uint32(5),'BlockType',struct('isSLSource',uint8(1),'isSLSink',uint8(1),'isHWSource',uint8(0),'isHWSink',uint8(0),'isSetup',uint8(0),'isInline',uint8(1),'isNonInline',uint8(0),'isInterrupt',uint8(0),'isChannelwise',uint8(0)),'IOBoardType','RTICAN','UnitType','MESSAGE','Identifier','RX','DialogType','MSVC','BlockSet','RTICAN','SlaveProcessor','CAN'))  RTIBlockInterface=struct('OutputPortsWidth',int32([1 1 1 1 1 1 1]),'OutputPortsActive',[1 1 1 1 1 1 1],'OutputPortsName',{{'Mux','state_bits','Message_nr','t_Value_highest','MidHigh','MidLow','Lowest'}},'OutputPortsDataType',{{'SS_UINT8','SS_UINT8','SS_UINT8','SS_UINT8','SS_UINT8','SS_UINT8','SS_UINT8'}},'OutputPortsLabel',{{'Mux','state_bits','Message_nr','t_Value_highest','MidHigh','MidLow','Lowest'}},'OutputPortsLabelMode','ON','InputPortsWidth',int32(0),'InputPortsActive',0,'DialogFcn','rtican_message_interface_gui','BlockDisplay',{{'','center'}},'IconTransparency','on','ParameterTunableNames',{{}},'InitLevel',3,'BlockName',struct('Token',{{'IVt_msg_result_t'}}),'SampleTime',{{-1}},'TriggerPort',{{'none'}},'EnablePort',{{'none'}})  RTIBlockParameters=struct('BoardTypeNo',{{1,'OFF',[]}},'BoardNo',{{2,'ON',[1 16]}},'ChannelNo',{{2,'ON',[1 2]}},'Parameters',{{struct('DataFileSupport',struct('DataFileSelectedMaster',0,'DataFileSelectedLocal',0,'DataFileName',['<no datafile support>|'],'DataFileDate','','SelectedFile',['<no file selected>']),'Options',struct('StatusSelected',0,'TimeSelected',0,'DeltaTimeSelected',0,'BytePortSelected',0,'MessageLengthSelected',0,'TriggerPort',struct('Selected',0,'TriggerType',0),'UserCoding',struct('Selected',0,'InterfaceFile','UserDecodingFile','FcnName','UserDecodeFcn','InportSelected',0,'InportWidth',1,'OutportSelected',0,'OutportWidth',1),'EnablePortSelected',0,'SignalOnPortnameSelected',1,'UseRXService',0),'Message',struct('MsgOnBlocknameSelected',1,'MsgName','IVt_msg_result_t','MsgIdFormat',0,'MsgId',1317,'MsgLength',6,'NumSignals',7,'SampleTime',-1,'Signal',struct('SgnName',{'Mux','state_bits','Message_nr','t_Value_highest','MidHigh','MidLow','Lowest'},'SgnStartBit',{0,8,12,16,24,32,40},'SgnLength',{8,4,4,8,8,8,8},'SgnType',{0,0,0,0,0,0,0},'ModeValue',{-1,-1,-1,-1,-1,-1,-1},'DataType',{0,0,0,0,0,0,0},'ByteLayout',{1,1,1,1,1,1,1},'Factor',{1,1,1,1,1,1,1},'Offset',{0,0,0,0,0,0,0},'SgnComment',{{''},{''},{''},{''},{''},{''},{''}},'SgnUnit',{'','','','','','',''},'Min',{0,0,0,0,0,0,0},'Max',{255,255,255,255,255,255,255},'SLDataType',{'SS_UINT8','SS_UINT8','SS_UINT8','SS_UINT8','SS_UINT8','SS_UINT8','SS_UINT8'}),'MsgIdNumFormat',1,'MsgComment',{{''}}),'Version',1.2,'general',struct('isFromLib',0)),'OFF',[]}},'GroupId',{{struct('Group',{{'RTICAN'}},'No',4,'Behavior',{{'NAMECHANGE'}},'BlockType',{{'SINK'}},'NameChangeFlag',0),'OFF',[]}},'SFcnRTICANMessage',{{struct('MsgType','RX','SFcnPortType','Scalar','MsgName','IVt_msg_result_t','MsgIdFormat','STD','MsgId',1317,'MsgLength',6,'NumSignals',7,'SampleTime',-1,'Signal',struct('SgnName',{'Mux','state_bits','Message_nr','t_Value_highest','MidHigh','MidLow','Lowest'},'SgnStartBit',{0,8,12,16,24,32,40},'SgnLength',{8,4,4,8,8,8,8},'SgnType',{'standard','standard','standard','standard','standard','standard','standard'},'ModeValue',{-1,-1,-1,-1,-1,-1,-1},'DataType',{['unsigned int'],['unsigned int'],['unsigned int'],['unsigned int'],['unsigned int'],['unsigned int'],['unsigned int']},'ByteLayout',{['big endian'],['big endian'],['big endian'],['big endian'],['big endian'],['big endian'],['big endian']},'Factor',{1,1,1,1,1,1,1},'Offset',{0,0,0,0,0,0,0},'SLDataType',{'SS_UINT8','SS_UINT8','SS_UINT8','SS_UINT8','SS_UINT8','SS_UINT8','SS_UINT8'}),'StatusSelected','no','TimeSelected','no','DeltaTimeSelected','no','BytePortSelected','no','MessageLengthSelected','no','TriggerPort',struct('Selected','no','TriggerType',0),'UserCoding',struct('Selected','no','InterfaceFile','UserDecodingFile','FcnName','UserDecodeFcn','InportSelected','no','InportWidth',1,'OutportSelected','no','OutportWidth',1),'EnablePortSelected','no','UseRXService','no','BoardType','DS1','BoardNo',2,'ControllerNo',2),'OFF',[]}},'TLCFileName',{{'rtican_rx_message','OFF',[]}})  RTISFcnParameters=struct('SFcnRTICANMessage','struct','TLCFileName','char')  RTIBlockParaDefault=struct('BoardTypeNo',4302,'BoardNo',1,'ChannelNo',1,'Parameters',struct('DataFileSupport',struct('DataFileSelectedMaster',0,'DataFileSelectedLocal',0,'DataFileName','','DataFileDate','','SelectedFile',['<no file selected>']),'Options',struct('StatusSelected',1,'TimeSelected',1,'DeltaTimeSelected',1,'BytePortSelected',0,'MessageLengthSelected',0,'TriggerPort',struct('Selected',0,'TriggerType','rising'),'UserCoding',struct('Selected',0,'InterfaceFile','UserDecodingFile','FcnName','UserDecodeFcn','InportSelected',0,'InportWidth',1,'OutportSelected',0,'OutportWidth',1),'EnablePortSelected',0,'SignalOnPortnameSelected',1,'UseRXService',0),'Message',struct('MsgOnBlocknameSelected',0,'MsgName',['RX Message'],'MsgIdFormat',0,'MsgId',100,'MsgLength',8,'NumSignals',1,'SampleTime',-1,'Signal',struct('SgnName',['RX signal'],'SgnStartBit',0,'SgnLength',8,'SgnType',0,'ModeValue',-1,'DataType',0,'SLDataType','SS_DOUBLE','ByteLayout',0,'Factor',1,'Offset',0,'Min',0,'Max',255,'SgnComment',{{}},'SgnUnit',''),'MsgIdNumFormat',0,'MsgComment',{{''}}),'Version',1.2,'general',struct('isFromLib',1)),'GroupId',struct('Group',{{'RTICAN'}},'No',1,'Behavior',{{'NAMECHANGE'}},'BlockType',{{'SINK'}},'NameChangeFlag',0),'SFcnRTICANMessage',struct('MsgType','RX','MsgName',['RX Message'],'MsgIdFormat','STD','MsgId',100,'MsgLength',8,'NumSignals',1,'SampleTime',-1,'Signal',struct('SgnName',['RX signal'],'SgnStartBit',0,'SgnLength',8,'SgnType','standard','ModeValue',-1,'DataType',['unsigned int'],'ByteLayout',['little endian'],'SLDataType','SS_DOUBLE','Factor',1,'Offset',0),'StatusSelected','yes','TimeSelected','yes','DeltaTimeSelected','yes','BytePortSelected','no','MessageLengthSelected','no','EnablePortSelected','no','UserCoding',struct('Selected','no','InterfaceFile','UserDecodingFile','FcnName','UserDecodeFcn','InportSelected','no','InportWidth',1,'OutportSelected','no','OutportWidth',1),'TriggerPort',struct('Selected','no','TriggerType','rising'),'UseRXService','no','BoardType','DS4302','BoardNo',1,'ControllerNo',1,'SFcnPortType','Scalar'),'TLCFileName','rtican_rx_message')
      settings: AttributesFormatString=Group Id: RTICAN4\n
  IVt_msg_result_u1 : rtican/RTICAN Receive (RX)   Reserved1=[]  Reserved2=[]  Reserved3=[]  Reserved4=[]  SfcnMessage=[]  Msg_Struct=[]  BoardTypeNo=[]  BoardNo=[]  ChannelNo=[]  Parameters=[]  DialogFcn=[]  UnitName=[]  Revision=[]  UnitValues=[]  DSProperties=struct('RTI',struct('Version',uint32(5),'BlockType',struct('isSLSource',uint8(1),'isSLSink',uint8(1),'isHWSource',uint8(0),'isHWSink',uint8(0),'isSetup',uint8(0),'isInline',uint8(1),'isNonInline',uint8(0),'isInterrupt',uint8(0),'isChannelwise',uint8(0)),'IOBoardType','RTICAN','UnitType','MESSAGE','Identifier','RX','DialogType','MSVC','BlockSet','RTICAN','SlaveProcessor','CAN'))  RTIBlockInterface=struct('OutputPortsWidth',int32([1 1 1 1 1 1 1]),'OutputPortsActive',[1 1 1 1 1 1 1],'OutputPortsName',{{'Mux','state_bits','Message_nr','V1_Value_highest','MidHigh','MidLow','Lowest'}},'OutputPortsDataType',{{'SS_UINT8','SS_UINT8','SS_UINT8','SS_UINT8','SS_UINT8','SS_UINT8','SS_UINT8'}},'OutputPortsLabel',{{'Mux','state_bits','Message_nr','V1_Value_highest','MidHigh','MidLow','Lowest'}},'OutputPortsLabelMode','ON','InputPortsWidth',int32(0),'InputPortsActive',0,'DialogFcn','rtican_message_interface_gui','BlockDisplay',{{'','center'}},'IconTransparency','on','ParameterTunableNames',{{}},'InitLevel',3,'BlockName',struct('Token',{{'IVt_msg_result_u1'}}),'SampleTime',{{-1}},'TriggerPort',{{'none'}},'EnablePort',{{'none'}})  RTIBlockParameters=struct('BoardTypeNo',{{1,'OFF',[]}},'BoardNo',{{2,'ON',[1 16]}},'ChannelNo',{{2,'ON',[1 2]}},'Parameters',{{struct('DataFileSupport',struct('DataFileSelectedMaster',0,'DataFileSelectedLocal',0,'DataFileName',['<no datafile support>|'],'DataFileDate','','SelectedFile',['<no file selected>']),'Options',struct('StatusSelected',0,'TimeSelected',0,'DeltaTimeSelected',0,'BytePortSelected',0,'MessageLengthSelected',0,'TriggerPort',struct('Selected',0,'TriggerType',0),'UserCoding',struct('Selected',0,'InterfaceFile','UserDecodingFile','FcnName','UserDecodeFcn','InportSelected',0,'InportWidth',1,'OutportSelected',0,'OutportWidth',1),'EnablePortSelected',0,'SignalOnPortnameSelected',1,'UseRXService',0),'Message',struct('MsgOnBlocknameSelected',1,'MsgName','IVt_msg_result_u1','MsgIdFormat',0,'MsgId',1314,'MsgLength',6,'NumSignals',7,'SampleTime',-1,'Signal',struct('SgnName',{'Mux','state_bits','Message_nr','V1_Value_highest','MidHigh','MidLow','Lowest'},'SgnStartBit',{0,8,12,16,24,32,40},'SgnLength',{8,4,4,8,8,8,8},'SgnType',{0,0,0,0,0,0,0},'ModeValue',{-1,-1,-1,-1,-1,-1,-1},'DataType',{0,0,0,0,0,0,0},'ByteLayout',{1,1,1,1,1,1,1},'Factor',{1,1,1,1,1,1,1},'Offset',{0,0,0,0,0,0,0},'SgnComment',{{''},{''},{''},{''},{''},{''},{''}},'SgnUnit',{'','','','','','',''},'Min',{0,0,0,0,0,0,0},'Max',{255,255,255,255,255,255,255},'SLDataType',{'SS_UINT8','SS_UINT8','SS_UINT8','SS_UINT8','SS_UINT8','SS_UINT8','SS_UINT8'}),'MsgIdNumFormat',1,'MsgComment',{{''}}),'Version',1.2,'general',struct('isFromLib',0)),'OFF',[]}},'GroupId',{{struct('Group',{{'RTICAN'}},'No',4,'Behavior',{{'NAMECHANGE'}},'BlockType',{{'SINK'}},'NameChangeFlag',0),'OFF',[]}},'SFcnRTICANMessage',{{struct('MsgType','RX','SFcnPortType','Scalar','MsgName','IVt_msg_result_u1','MsgIdFormat','STD','MsgId',1314,'MsgLength',6,'NumSignals',7,'SampleTime',-1,'Signal',struct('SgnName',{'Mux','state_bits','Message_nr','V1_Value_highest','MidHigh','MidLow','Lowest'},'SgnStartBit',{0,8,12,16,24,32,40},'SgnLength',{8,4,4,8,8,8,8},'SgnType',{'standard','standard','standard','standard','standard','standard','standard'},'ModeValue',{-1,-1,-1,-1,-1,-1,-1},'DataType',{['unsigned int'],['unsigned int'],['unsigned int'],['unsigned int'],['unsigned int'],['unsigned int'],['unsigned int']},'ByteLayout',{['big endian'],['big endian'],['big endian'],['big endian'],['big endian'],['big endian'],['big endian']},'Factor',{1,1,1,1,1,1,1},'Offset',{0,0,0,0,0,0,0},'SLDataType',{'SS_UINT8','SS_UINT8','SS_UINT8','SS_UINT8','SS_UINT8','SS_UINT8','SS_UINT8'}),'StatusSelected','no','TimeSelected','no','DeltaTimeSelected','no','BytePortSelected','no','MessageLengthSelected','no','TriggerPort',struct('Selected','no','TriggerType',0),'UserCoding',struct('Selected','no','InterfaceFile','UserDecodingFile','FcnName','UserDecodeFcn','InportSelected','no','InportWidth',1,'OutportSelected','no','OutportWidth',1),'EnablePortSelected','no','UseRXService','no','BoardType','DS1','BoardNo',2,'ControllerNo',2),'OFF',[]}},'TLCFileName',{{'rtican_rx_message','OFF',[]}})  RTISFcnParameters=struct('SFcnRTICANMessage','struct','TLCFileName','char')  RTIBlockParaDefault=struct('BoardTypeNo',4302,'BoardNo',1,'ChannelNo',1,'Parameters',struct('DataFileSupport',struct('DataFileSelectedMaster',0,'DataFileSelectedLocal',0,'DataFileName','','DataFileDate','','SelectedFile',['<no file selected>']),'Options',struct('StatusSelected',1,'TimeSelected',1,'DeltaTimeSelected',1,'BytePortSelected',0,'MessageLengthSelected',0,'TriggerPort',struct('Selected',0,'TriggerType','rising'),'UserCoding',struct('Selected',0,'InterfaceFile','UserDecodingFile','FcnName','UserDecodeFcn','InportSelected',0,'InportWidth',1,'OutportSelected',0,'OutportWidth',1),'EnablePortSelected',0,'SignalOnPortnameSelected',1,'UseRXService',0),'Message',struct('MsgOnBlocknameSelected',0,'MsgName',['RX Message'],'MsgIdFormat',0,'MsgId',100,'MsgLength',8,'NumSignals',1,'SampleTime',-1,'Signal',struct('SgnName',['RX signal'],'SgnStartBit',0,'SgnLength',8,'SgnType',0,'ModeValue',-1,'DataType',0,'SLDataType','SS_DOUBLE','ByteLayout',0,'Factor',1,'Offset',0,'Min',0,'Max',255,'SgnComment',{{}},'SgnUnit',''),'MsgIdNumFormat',0,'MsgComment',{{''}}),'Version',1.2,'general',struct('isFromLib',1)),'GroupId',struct('Group',{{'RTICAN'}},'No',1,'Behavior',{{'NAMECHANGE'}},'BlockType',{{'SINK'}},'NameChangeFlag',0),'SFcnRTICANMessage',struct('MsgType','RX','MsgName',['RX Message'],'MsgIdFormat','STD','MsgId',100,'MsgLength',8,'NumSignals',1,'SampleTime',-1,'Signal',struct('SgnName',['RX signal'],'SgnStartBit',0,'SgnLength',8,'SgnType','standard','ModeValue',-1,'DataType',['unsigned int'],'ByteLayout',['little endian'],'SLDataType','SS_DOUBLE','Factor',1,'Offset',0),'StatusSelected','yes','TimeSelected','yes','DeltaTimeSelected','yes','BytePortSelected','no','MessageLengthSelected','no','EnablePortSelected','no','UserCoding',struct('Selected','no','InterfaceFile','UserDecodingFile','FcnName','UserDecodeFcn','InportSelected','no','InportWidth',1,'OutportSelected','no','OutportWidth',1),'TriggerPort',struct('Selected','no','TriggerType','rising'),'UseRXService','no','BoardType','DS4302','BoardNo',1,'ControllerNo',1,'SFcnPortType','Scalar'),'TLCFileName','rtican_rx_message')
      settings: AttributesFormatString=Group Id: RTICAN4\n
  IVt_msg_result_u2 : rtican/RTICAN Receive (RX)   Reserved1=[]  Reserved2=[]  Reserved3=[]  Reserved4=[]  SfcnMessage=[]  Msg_Struct=[]  BoardTypeNo=[]  BoardNo=[]  ChannelNo=[]  Parameters=[]  DialogFcn=[]  UnitName=[]  Revision=[]  UnitValues=[]  DSProperties=struct('RTI',struct('Version',uint32(5),'BlockType',struct('isSLSource',uint8(1),'isSLSink',uint8(1),'isHWSource',uint8(0),'isHWSink',uint8(0),'isSetup',uint8(0),'isInline',uint8(1),'isNonInline',uint8(0),'isInterrupt',uint8(0),'isChannelwise',uint8(0)),'IOBoardType','RTICAN','UnitType','MESSAGE','Identifier','RX','DialogType','MSVC','BlockSet','RTICAN','SlaveProcessor','CAN'))  RTIBlockInterface=struct('OutputPortsWidth',int32([1 1 1 1 1 1 1]),'OutputPortsActive',[1 1 1 1 1 1 1],'OutputPortsName',{{'Mux','state_bits','Message_nr','V2_Value_highest','MidHigh','MidLow','Lowest'}},'OutputPortsDataType',{{'SS_UINT8','SS_UINT8','SS_UINT8','SS_UINT8','SS_UINT8','SS_UINT8','SS_UINT8'}},'OutputPortsLabel',{{'Mux','state_bits','Message_nr','V2_Value_highest','MidHigh','MidLow','Lowest'}},'OutputPortsLabelMode','ON','InputPortsWidth',int32(0),'InputPortsActive',0,'DialogFcn','rtican_message_interface_gui','BlockDisplay',{{'','center'}},'IconTransparency','on','ParameterTunableNames',{{}},'InitLevel',3,'BlockName',struct('Token',{{'IVt_msg_result_u2'}}),'SampleTime',{{-1}},'TriggerPort',{{'none'}},'EnablePort',{{'none'}})  RTIBlockParameters=struct('BoardTypeNo',{{1,'OFF',[]}},'BoardNo',{{2,'ON',[1 16]}},'ChannelNo',{{2,'ON',[1 2]}},'Parameters',{{struct('DataFileSupport',struct('DataFileSelectedMaster',0,'DataFileSelectedLocal',0,'DataFileName',['<no datafile support>|'],'DataFileDate','','SelectedFile',['<no file selected>']),'Options',struct('StatusSelected',0,'TimeSelected',0,'DeltaTimeSelected',0,'BytePortSelected',0,'MessageLengthSelected',0,'TriggerPort',struct('Selected',0,'TriggerType',0),'UserCoding',struct('Selected',0,'InterfaceFile','UserDecodingFile','FcnName','UserDecodeFcn','InportSelected',0,'InportWidth',1,'OutportSelected',0,'OutportWidth',1),'EnablePortSelected',0,'SignalOnPortnameSelected',1,'UseRXService',0),'Message',struct('MsgOnBlocknameSelected',1,'MsgName','IVt_msg_result_u2','MsgIdFormat',0,'MsgId',1315,'MsgLength',6,'NumSignals',7,'SampleTime',-1,'Signal',struct('SgnName',{'Mux','state_bits','Message_nr','V2_Value_highest','MidHigh','MidLow','Lowest'},'SgnStartBit',{0,8,12,16,24,32,40},'SgnLength',{8,4,4,8,8,8,8},'SgnType',{0,0,0,0,0,0,0},'ModeValue',{-1,-1,-1,-1,-1,-1,-1},'DataType',{0,0,0,0,0,0,0},'ByteLayout',{1,1,1,1,1,1,1},'Factor',{1,1,1,1,1,1,1},'Offset',{0,0,0,0,0,0,0},'SgnComment',{{''},{''},{''},{''},{''},{''},{''}},'SgnUnit',{'','','','','','',''},'Min',{0,0,0,0,0,0,0},'Max',{255,255,255,255,255,255,255},'SLDataType',{'SS_UINT8','SS_UINT8','SS_UINT8','SS_UINT8','SS_UINT8','SS_UINT8','SS_UINT8'}),'MsgIdNumFormat',1,'MsgComment',{{''}}),'Version',1.2,'general',struct('isFromLib',0)),'OFF',[]}},'GroupId',{{struct('Group',{{'RTICAN'}},'No',4,'Behavior',{{'NAMECHANGE'}},'BlockType',{{'SINK'}},'NameChangeFlag',0),'OFF',[]}},'SFcnRTICANMessage',{{struct('MsgType','RX','SFcnPortType','Scalar','MsgName','IVt_msg_result_u2','MsgIdFormat','STD','MsgId',1315,'MsgLength',6,'NumSignals',7,'SampleTime',-1,'Signal',struct('SgnName',{'Mux','state_bits','Message_nr','V2_Value_highest','MidHigh','MidLow','Lowest'},'SgnStartBit',{0,8,12,16,24,32,40},'SgnLength',{8,4,4,8,8,8,8},'SgnType',{'standard','standard','standard','standard','standard','standard','standard'},'ModeValue',{-1,-1,-1,-1,-1,-1,-1},'DataType',{['unsigned int'],['unsigned int'],['unsigned int'],['unsigned int'],['unsigned int'],['unsigned int'],['unsigned int']},'ByteLayout',{['big endian'],['big endian'],['big endian'],['big endian'],['big endian'],['big endian'],['big endian']},'Factor',{1,1,1,1,1,1,1},'Offset',{0,0,0,0,0,0,0},'SLDataType',{'SS_UINT8','SS_UINT8','SS_UINT8','SS_UINT8','SS_UINT8','SS_UINT8','SS_UINT8'}),'StatusSelected','no','TimeSelected','no','DeltaTimeSelected','no','BytePortSelected','no','MessageLengthSelected','no','TriggerPort',struct('Selected','no','TriggerType',0),'UserCoding',struct('Selected','no','InterfaceFile','UserDecodingFile','FcnName','UserDecodeFcn','InportSelected','no','InportWidth',1,'OutportSelected','no','OutportWidth',1),'EnablePortSelected','no','UseRXService','no','BoardType','DS1','BoardNo',2,'ControllerNo',2),'OFF',[]}},'TLCFileName',{{'rtican_rx_message','OFF',[]}})  RTISFcnParameters=struct('SFcnRTICANMessage','struct','TLCFileName','char')  RTIBlockParaDefault=struct('BoardTypeNo',4302,'BoardNo',1,'ChannelNo',1,'Parameters',struct('DataFileSupport',struct('DataFileSelectedMaster',0,'DataFileSelectedLocal',0,'DataFileName','','DataFileDate','','SelectedFile',['<no file selected>']),'Options',struct('StatusSelected',1,'TimeSelected',1,'DeltaTimeSelected',1,'BytePortSelected',0,'MessageLengthSelected',0,'TriggerPort',struct('Selected',0,'TriggerType','rising'),'UserCoding',struct('Selected',0,'InterfaceFile','UserDecodingFile','FcnName','UserDecodeFcn','InportSelected',0,'InportWidth',1,'OutportSelected',0,'OutportWidth',1),'EnablePortSelected',0,'SignalOnPortnameSelected',1,'UseRXService',0),'Message',struct('MsgOnBlocknameSelected',0,'MsgName',['RX Message'],'MsgIdFormat',0,'MsgId',100,'MsgLength',8,'NumSignals',1,'SampleTime',-1,'Signal',struct('SgnName',['RX signal'],'SgnStartBit',0,'SgnLength',8,'SgnType',0,'ModeValue',-1,'DataType',0,'SLDataType','SS_DOUBLE','ByteLayout',0,'Factor',1,'Offset',0,'Min',0,'Max',255,'SgnComment',{{}},'SgnUnit',''),'MsgIdNumFormat',0,'MsgComment',{{''}}),'Version',1.2,'general',struct('isFromLib',1)),'GroupId',struct('Group',{{'RTICAN'}},'No',1,'Behavior',{{'NAMECHANGE'}},'BlockType',{{'SINK'}},'NameChangeFlag',0),'SFcnRTICANMessage',struct('MsgType','RX','MsgName',['RX Message'],'MsgIdFormat','STD','MsgId',100,'MsgLength',8,'NumSignals',1,'SampleTime',-1,'Signal',struct('SgnName',['RX signal'],'SgnStartBit',0,'SgnLength',8,'SgnType','standard','ModeValue',-1,'DataType',['unsigned int'],'ByteLayout',['little endian'],'SLDataType','SS_DOUBLE','Factor',1,'Offset',0),'StatusSelected','yes','TimeSelected','yes','DeltaTimeSelected','yes','BytePortSelected','no','MessageLengthSelected','no','EnablePortSelected','no','UserCoding',struct('Selected','no','InterfaceFile','UserDecodingFile','FcnName','UserDecodeFcn','InportSelected','no','InportWidth',1,'OutportSelected','no','OutportWidth',1),'TriggerPort',struct('Selected','no','TriggerType','rising'),'UseRXService','no','BoardType','DS4302','BoardNo',1,'ControllerNo',1,'SFcnPortType','Scalar'),'TLCFileName','rtican_rx_message')
      settings: AttributesFormatString=Group Id: RTICAN4\n
  IVt_msg_result_u3 : rtican/RTICAN Receive (RX)   Reserved1=[]  Reserved2=[]  Reserved3=[]  Reserved4=[]  SfcnMessage=[]  Msg_Struct=[]  BoardTypeNo=[]  BoardNo=[]  ChannelNo=[]  Parameters=[]  DialogFcn=[]  UnitName=[]  Revision=[]  UnitValues=[]  DSProperties=struct('RTI',struct('Version',uint32(5),'BlockType',struct('isSLSource',uint8(1),'isSLSink',uint8(1),'isHWSource',uint8(0),'isHWSink',uint8(0),'isSetup',uint8(0),'isInline',uint8(1),'isNonInline',uint8(0),'isInterrupt',uint8(0),'isChannelwise',uint8(0)),'IOBoardType','RTICAN','UnitType','MESSAGE','Identifier','RX','DialogType','MSVC','BlockSet','RTICAN','SlaveProcessor','CAN'))  RTIBlockInterface=struct('OutputPortsWidth',int32([1 1 1 1 1 1 1]),'OutputPortsActive',[1 1 1 1 1 1 1],'OutputPortsName',{{'Mux','state_bits','Message_nr','V3_Value_high','MidHigh','MidLow','Lowest'}},'OutputPortsDataType',{{'SS_UINT8','SS_UINT8','SS_UINT8','SS_UINT8','SS_UINT8','SS_UINT8','SS_UINT8'}},'OutputPortsLabel',{{'Mux','state_bits','Message_nr','V3_Value_high','MidHigh','MidLow','Lowest'}},'OutputPortsLabelMode','ON','InputPortsWidth',int32(0),'InputPortsActive',0,'DialogFcn','rtican_message_interface_gui','BlockDisplay',{{'','center'}},'IconTransparency','on','ParameterTunableNames',{{}},'InitLevel',3,'BlockName',struct('Token',{{'IVt_msg_result_u3'}}),'SampleTime',{{-1}},'TriggerPort',{{'none'}},'EnablePort',{{'none'}})  RTIBlockParameters=struct('BoardTypeNo',{{1,'OFF',[]}},'BoardNo',{{2,'ON',[1 16]}},'ChannelNo',{{2,'ON',[1 2]}},'Parameters',{{struct('DataFileSupport',struct('DataFileSelectedMaster',0,'DataFileSelectedLocal',0,'DataFileName',['<no datafile support>|'],'DataFileDate','','SelectedFile',['<no file selected>']),'Options',struct('StatusSelected',0,'TimeSelected',0,'DeltaTimeSelected',0,'BytePortSelected',0,'MessageLengthSelected',0,'TriggerPort',struct('Selected',0,'TriggerType',0),'UserCoding',struct('Selected',0,'InterfaceFile','UserDecodingFile','FcnName','UserDecodeFcn','InportSelected',0,'InportWidth',1,'OutportSelected',0,'OutportWidth',1),'EnablePortSelected',0,'SignalOnPortnameSelected',1,'UseRXService',0),'Message',struct('MsgOnBlocknameSelected',1,'MsgName','IVt_msg_result_u3','MsgIdFormat',0,'MsgId',1316,'MsgLength',6,'NumSignals',7,'SampleTime',-1,'Signal',struct('SgnName',{'Mux','state_bits','Message_nr','V3_Value_high','MidHigh','MidLow','Lowest'},'SgnStartBit',{0,8,12,16,24,32,40},'SgnLength',{8,4,4,8,8,8,8},'SgnType',{0,0,0,0,0,0,0},'ModeValue',{-1,-1,-1,-1,-1,-1,-1},'DataType',{0,0,0,0,0,0,0},'ByteLayout',{1,1,1,1,1,1,1},'Factor',{1,1,1,1,1,1,1},'Offset',{0,0,0,0,0,0,0},'SgnComment',{{''},{''},{''},{''},{''},{''},{''}},'SgnUnit',{'','','','','','',''},'Min',{0,0,0,0,0,0,0},'Max',{255,255,255,255,255,255,255},'SLDataType',{'SS_UINT8','SS_UINT8','SS_UINT8','SS_UINT8','SS_UINT8','SS_UINT8','SS_UINT8'}),'MsgIdNumFormat',1,'MsgComment',{{''}}),'Version',1.2,'general',struct('isFromLib',0)),'OFF',[]}},'GroupId',{{struct('Group',{{'RTICAN'}},'No',4,'Behavior',{{'NAMECHANGE'}},'BlockType',{{'SINK'}},'NameChangeFlag',0),'OFF',[]}},'SFcnRTICANMessage',{{struct('MsgType','RX','SFcnPortType','Scalar','MsgName','IVt_msg_result_u3','MsgIdFormat','STD','MsgId',1316,'MsgLength',6,'NumSignals',7,'SampleTime',-1,'Signal',struct('SgnName',{'Mux','state_bits','Message_nr','V3_Value_high','MidHigh','MidLow','Lowest'},'SgnStartBit',{0,8,12,16,24,32,40},'SgnLength',{8,4,4,8,8,8,8},'SgnType',{'standard','standard','standard','standard','standard','standard','standard'},'ModeValue',{-1,-1,-1,-1,-1,-1,-1},'DataType',{['unsigned int'],['unsigned int'],['unsigned int'],['unsigned int'],['unsigned int'],['unsigned int'],['unsigned int']},'ByteLayout',{['big endian'],['big endian'],['big endian'],['big endian'],['big endian'],['big endian'],['big endian']},'Factor',{1,1,1,1,1,1,1},'Offset',{0,0,0,0,0,0,0},'SLDataType',{'SS_UINT8','SS_UINT8','SS_UINT8','SS_UINT8','SS_UINT8','SS_UINT8','SS_UINT8'}),'StatusSelected','no','TimeSelected','no','DeltaTimeSelected','no','BytePortSelected','no','MessageLengthSelected','no','TriggerPort',struct('Selected','no','TriggerType',0),'UserCoding',struct('Selected','no','InterfaceFile','UserDecodingFile','FcnName','UserDecodeFcn','InportSelected','no','InportWidth',1,'OutportSelected','no','OutportWidth',1),'EnablePortSelected','no','UseRXService','no','BoardType','DS1','BoardNo',2,'ControllerNo',2),'OFF',[]}},'TLCFileName',{{'rtican_rx_message','OFF',[]}})  RTISFcnParameters=struct('SFcnRTICANMessage','struct','TLCFileName','char')  RTIBlockParaDefault=struct('BoardTypeNo',4302,'BoardNo',1,'ChannelNo',1,'Parameters',struct('DataFileSupport',struct('DataFileSelectedMaster',0,'DataFileSelectedLocal',0,'DataFileName','','DataFileDate','','SelectedFile',['<no file selected>']),'Options',struct('StatusSelected',1,'TimeSelected',1,'DeltaTimeSelected',1,'BytePortSelected',0,'MessageLengthSelected',0,'TriggerPort',struct('Selected',0,'TriggerType','rising'),'UserCoding',struct('Selected',0,'InterfaceFile','UserDecodingFile','FcnName','UserDecodeFcn','InportSelected',0,'InportWidth',1,'OutportSelected',0,'OutportWidth',1),'EnablePortSelected',0,'SignalOnPortnameSelected',1,'UseRXService',0),'Message',struct('MsgOnBlocknameSelected',0,'MsgName',['RX Message'],'MsgIdFormat',0,'MsgId',100,'MsgLength',8,'NumSignals',1,'SampleTime',-1,'Signal',struct('SgnName',['RX signal'],'SgnStartBit',0,'SgnLength',8,'SgnType',0,'ModeValue',-1,'DataType',0,'SLDataType','SS_DOUBLE','ByteLayout',0,'Factor',1,'Offset',0,'Min',0,'Max',255,'SgnComment',{{}},'SgnUnit',''),'MsgIdNumFormat',0,'MsgComment',{{''}}),'Version',1.2,'general',struct('isFromLib',1)),'GroupId',struct('Group',{{'RTICAN'}},'No',1,'Behavior',{{'NAMECHANGE'}},'BlockType',{{'SINK'}},'NameChangeFlag',0),'SFcnRTICANMessage',struct('MsgType','RX','MsgName',['RX Message'],'MsgIdFormat','STD','MsgId',100,'MsgLength',8,'NumSignals',1,'SampleTime',-1,'Signal',struct('SgnName',['RX signal'],'SgnStartBit',0,'SgnLength',8,'SgnType','standard','ModeValue',-1,'DataType',['unsigned int'],'ByteLayout',['little endian'],'SLDataType','SS_DOUBLE','Factor',1,'Offset',0),'StatusSelected','yes','TimeSelected','yes','DeltaTimeSelected','yes','BytePortSelected','no','MessageLengthSelected','no','EnablePortSelected','no','UserCoding',struct('Selected','no','InterfaceFile','UserDecodingFile','FcnName','UserDecodeFcn','InportSelected','no','InportWidth',1,'OutportSelected','no','OutportWidth',1),'TriggerPort',struct('Selected','no','TriggerType','rising'),'UseRXService','no','BoardType','DS4302','BoardNo',1,'ControllerNo',1,'SFcnPortType','Scalar'),'TLCFileName','rtican_rx_message')
      settings: AttributesFormatString=Group Id: RTICAN4\n
  MATLAB Function : MATLAB Function  TreatAsAtomicUnit=on
  parseAs : MATLAB Function  TreatAsAtomicUnit=on
  "parseCurrent " : MATLAB Function  TreatAsAtomicUnit=on
  parseEnergy : MATLAB Function  TreatAsAtomicUnit=on
  parseTemperature : MATLAB Function  TreatAsAtomicUnit=on
  parseVoltage1 : MATLAB Function  TreatAsAtomicUnit=on
  parseVoltage2 : MATLAB Function  TreatAsAtomicUnit=on
  parseVoltage3 : MATLAB Function  TreatAsAtomicUnit=on
  parseWh : MATLAB Function  TreatAsAtomicUnit=on
  "EM " : Outport
  wires:
  IVt_msg_result_I/1 -> "parseCurrent "/1(Mux)  "Mux"
  IVt_msg_result_I/2 -> "parseCurrent "/2(status)  "state_bits"
  IVt_msg_result_I/3 -> "parseCurrent "/3(messageNr)  "Message_nr"
  IVt_msg_result_u1/1 -> parseVoltage1/1(Mux)  "Mux"
  IVt_msg_result_u1/2 -> parseVoltage1/2(status)  "state_bits"
  IVt_msg_result_u1/3 -> parseVoltage1/3(messageNr)  "Message_nr"
  IVt_msg_result_Wh/1 -> parseWh/1(Mux)  "Mux"
  IVt_msg_result_Wh/2 -> parseWh/2(status)  "state_bits"
  IVt_msg_result_Wh/3 -> parseWh/3(messageNr)  "Message_nr"
  IVt_msg_result_AS/3 -> parseAs/3(messageNr)  "Message_nr"
  IVt_msg_result_AS/2 -> parseAs/2(status)  "state_bits"
  IVt_msg_result_AS/1 -> parseAs/1(Mux)  "Mux"
  IVt_msg_result_W/3 -> parseEnergy/3(messageNr)  "Message_nr"
  IVt_msg_result_W/2 -> parseEnergy/2(status)  "state_bits"
  IVt_msg_result_W/1 -> parseEnergy/1(Mux)  "Mux"
  IVt_msg_result_t1/1 -> parseTemperature/1(Mux)  "Mux"
  IVt_msg_result_t1/2 -> parseTemperature/2(status)  "state_bits"
  IVt_msg_result_t1/3 -> parseTemperature/3(messageNr)  "Message_nr"
  IVt_msg_result_u3/4 -> parseVoltage3/4(valueHighest)  "V3_Value_high"
  IVt_msg_result_u3/3 -> parseVoltage3/3(messageNr)  "Message_nr"
  IVt_msg_result_u3/2 -> parseVoltage3/2(status)  "state_bits"
  IVt_msg_result_u3/1 -> parseVoltage3/1(Mux)  "Mux"
  IVt_msg_result_u2/3 -> parseVoltage2/3(messageNr)  "Message_nr"
  IVt_msg_result_u2/2 -> parseVoltage2/2(status)  "state_bits"
  IVt_msg_result_u2/1 -> parseVoltage2/1(Mux)  "Mux"
  IVt_msg_response/8 -> MATLAB Function/8(response6)  "msg_response_data_6"
  IVt_msg_response/7 -> MATLAB Function/7(response5)  "msg_response_data_5"
  IVt_msg_response/6 -> MATLAB Function/6(response4)  "msg_response_data_4"
  IVt_msg_response/5 -> MATLAB Function/5(response3)  "msg_response_data_3"
  IVt_msg_response/4 -> MATLAB Function/4(response2)  "msg_response_data_2"
  IVt_msg_response/3 -> MATLAB Function/3(response1)  "msg_response_data_1"
  IVt_msg_response/2 -> MATLAB Function/2(response0)  "msg_response_data_0"
  IVt_msg_response/1 -> MATLAB Function/1(muxByte)  "msg_response_type"
  MATLAB Function/1(response) -> Bus Creator/1
  "parseCurrent "/1(current) -> Bus Creator/2
  parseVoltage1/1(voltage1) -> Bus Creator/3
  parseVoltage2/1(voltage2) -> Bus Creator/4
  parseVoltage3/1(voltage3) -> Bus Creator/5
  parseTemperature/1(temperature) -> Bus Creator/6
  parseEnergy/1(energy) -> Bus Creator/7
  parseAs/1(ampereSeconde) -> Bus Creator/8
  parseWh/1(wattHour) -> Bus Creator/9
  Bus Creator/1 -> "EM "/1
  IVt_msg_result_I/4 -> "parseCurrent "/4(valueHighest)  "Highest"
  IVt_msg_result_I/5 -> "parseCurrent "/5(valueMidHigh)  "MidHigh"
  IVt_msg_result_I/6 -> "parseCurrent "/6(valueMidLow)  "MidLow"
  IVt_msg_result_I/7 -> "parseCurrent "/7(valueLowest)  "Low"
  IVt_msg_result_u1/4 -> parseVoltage1/4(valueHighest)  "V1_Value_highest"
  IVt_msg_result_u1/5 -> parseVoltage1/5(valueMidHigh)  "MidHigh"
  IVt_msg_result_u1/6 -> parseVoltage1/6(valueMidLow)  "MidLow"
  IVt_msg_result_u1/7 -> parseVoltage1/7(valueLowest)  "Lowest"
  IVt_msg_result_u2/4 -> parseVoltage2/4(valueHighest)  "V2_Value_highest"
  IVt_msg_result_u2/5 -> parseVoltage2/5(valueMidHigh)  "MidHigh"
  IVt_msg_result_u2/6 -> parseVoltage2/6(valueMidLow)  "MidLow"
  IVt_msg_result_u2/7 -> parseVoltage2/7(valueLowest)  "Lowest"
  IVt_msg_result_u3/5 -> parseVoltage3/5(valueMidHigh)  "MidHigh"
  IVt_msg_result_u3/6 -> parseVoltage3/6(valueMidLow)  "MidLow"
  IVt_msg_result_u3/7 -> parseVoltage3/7(valueLowest)  "Lowest"
  IVt_msg_result_t1/4 -> parseTemperature/4(valueHighest)  "t_Value_highest"
  IVt_msg_result_t1/5 -> parseTemperature/5(valueMidHigh)  "MidHigh"
  IVt_msg_result_t1/6 -> parseTemperature/6(valueMidLow)  "MidLow"
  IVt_msg_result_t1/7 -> parseTemperature/7(valueLowest)  "Lowest"
  IVt_msg_result_W/4 -> parseEnergy/4(valueHighest)  "W_Value_highest"
  IVt_msg_result_W/5 -> parseEnergy/5(valueMidHigh)  "MidHigh"
  IVt_msg_result_W/6 -> parseEnergy/6(valueMidLow)  "MidLow"
  IVt_msg_result_W/7 -> parseEnergy/7(valueLowest)  "Lowest"
  IVt_msg_result_AS/4 -> parseAs/4(valueHighest)  "As_Value_highest"
  IVt_msg_result_AS/5 -> parseAs/5(valueMidHigh)  "MidHigh"
  IVt_msg_result_AS/6 -> parseAs/6(valueMidLow)  "MidLow"
  IVt_msg_result_AS/7 -> parseAs/7(valueLowest)  "Lowest"
  IVt_msg_result_Wh/4 -> parseWh/4(valueHighest)  "Wh_Value_highest"
  IVt_msg_result_Wh/5 -> parseWh/5(valueMidHigh)  "MidHigh"
  IVt_msg_result_Wh/6 -> parseWh/6(valueMidLow)  "MidLow"
  IVt_msg_result_Wh/7 -> parseWh/7(valueLowest)  "Lowest"
